simulink model "DATA_MTK_2"  (R2017a)
settings: Solver=ode1  StartTime=Times.Ts  StopTime=Times.Tsim  FixedStep=Times.Ts  RelTol=1e-3  EnableMultiTasking=on
values from neighbouring files (symbols this model uses):
  CL = 1    [Main_HydroVsData30min.m]
  WaveData = Init_waves_Data_V2(Time)    [Main_HydroVsData30min.m]
undefined symbols (not defined in the file or in its folder): Times, Turb, WEC
settings Model: Creator=FixnBock  LastModifiedBy=Temo
settings SolverCC: AlgebraicLoopSolver=LineSearch
settings DataIOCC: LimitDataPoints=on  SaveFormat=StructureWithTime
settings OptimizationCC: DefaultParameterBehavior=Inlined  LifeSpan=inf
settings DebuggingCC: AlgebraicLoopMsg=error  SFUnexpectedBacktrackingDiag=warning  SFNoUnconditionalDefaultTransitionDiag=warning  SFExecutionAtInitializationDiag=none
settings HardwareCC: ProdBitPerSizeT=32  ProdBitPerPtrDiffT=32  ProdWordSize=32  ProdHWDeviceType=Specified
settings ModelReferenceCC: PropagateSignalLabelsOutOfModel=off
settings RTWCC: TemplateMakefile=RTW.MSVCBuild  Description=Create Visual C/C++ Solution File for Simulink Coder
settings GRTTargetCC: TargetLangStandard=C89/C90 (ANSI)
settings ConfigComp: CovMetricSettings=dw  CovHtmlReporting=on  CovSaveCumulativeToWorkspaceVar=on  CovSaveSingleToWorkspaceVar=on  CovExternalEMLEnable=off

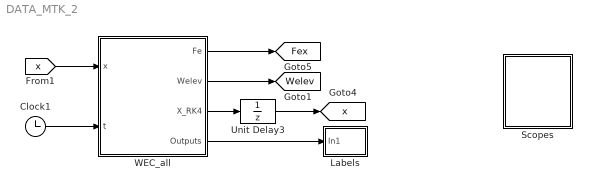
== system DATA_MTK_2 ==
  Clock1 : Clock
  Labels : Subsystem
  Scopes : Subsystem
  Unit Delay3 : UnitDelay  InitialCondition=WEC.X0  SampleTime=-1
  WEC_all : MATLAB Function  TreatAsAtomicUnit=on
  tag scope: Fex=global, Welev=global, x=global
  wires:
  Clock1/1 -> WEC_all/2(t)
  Unit Delay3/1 -> [x]
  [x] -> WEC_all/1(x)
  WEC_all/4(Outputs) -> Labels/1(In1)
  WEC_all/3(X_RK4) -> Unit Delay3/1
  WEC_all/1(Fe) -> [Fex]
  WEC_all/2(Welev) -> [Welev]

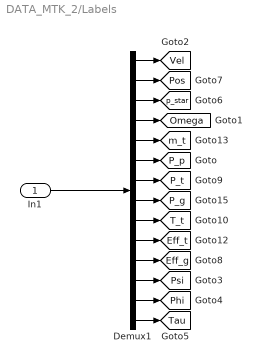
== system DATA_MTK_2/Labels ==
  In1 : Inport
  Demux1 : Demux  Outputs=14
  tag scope: Eff_g=global, Eff_t=global, Omega=global, P_g=global, P_p=global, P_t=global, Phi=global, Pos=global, Psi=global, T_t=global, Tau=global, Vel=global, m_t=global, p_star=global
  wires:
  Demux1/5 -> [m_t]
  Demux1/3 -> [p_star]
  Demux1/8 -> [P_g]
  Demux1/1 -> [Vel]
  Demux1/4 -> [Omega]
  Demux1/2 -> [Pos]
  Demux1/9 -> [T_t]
  Demux1/7 -> [P_t]
  Demux1/10 -> [Eff_t]
  Demux1/11 -> [Eff_g]
  Demux1/12 -> [Psi]
  Demux1/13 -> [Phi]
  Demux1/14 -> [Tau]
  Demux1/6 -> [P_p]
  In1/1 -> Demux1/1

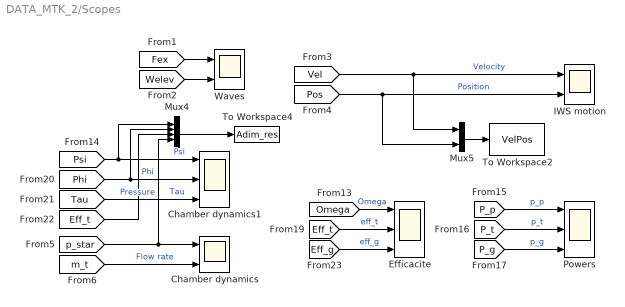
== system DATA_MTK_2/Scopes ==
  Chamber dynamics : Scope  NumInputPorts=2
  Chamber dynamics1 : Scope  NumInputPorts=3
  Efficacite : Scope  NumInputPorts=3
  IWS motion : Scope  NumInputPorts=2
  Mux4 : Mux
  Mux5 : Mux  Inputs=2
  Powers : Scope  NumInputPorts=3
  To Workspace2 : ToWorkspace  VariableName=VelPos  SampleTime=-1
      settings: Decimation=2
  To Workspace4 : ToWorkspace  VariableName=Adim_res  SampleTime=-1
      settings: Decimation=2
  Waves : Scope  NumInputPorts=2
  wires:
  [p_star] -> Mux4/4, Chamber dynamics/1  "Pressure"
  [m_t] -> Chamber dynamics/2  "Flow rate"
  [Welev] -> Waves/2
  [Fex] -> Waves/1
  [Psi] -> Mux4/1, Chamber dynamics1/1  "Psi"
  [Tau] -> Chamber dynamics1/3  "Tau"
  Mux4/1 -> To Workspace4/1
  [Eff_t] -> Mux4/3
  [Phi] -> Mux4/2, Chamber dynamics1/2  "Phi"
  [Vel] -> Mux5/1, IWS motion/1  "Velocity"
  [Pos] -> Mux5/2, IWS motion/2  "Position"
  Mux5/1 -> To Workspace2/1
  [Eff_t] -> Efficacite/2  "eff_t"
  [Eff_g] -> Efficacite/3  "eff_g"
  [P_g] -> Powers/3  "p_g"
  [P_t] -> Powers/2  "p_t"
  [P_p] -> Powers/1  "p_p"
  [Omega] -> Efficacite/1  "Omega"

== matlab function DATA_MTK_2/WEC_all ==
  data: x input size=24; t input; Fe output; WaveData parameter; WEC parameter; Turb parameter; Times parameter; CL parameter; Welev output; X_RK4 output; Outputs output
function [Fe,Welev,X_RK4,Outputs] = main(x,t,WaveData,WEC,Turb,Times,CL)

Ts = Times.Ts;

[Fexc,Welev] = resource(t,WaveData,WEC,Ts);
Fe = Fexc(3);

[X_RK4,Outputs] = fcn_rk4(t,x,Fexc,WEC,Turb,Ts,CL,Times);

end

function [Fe,welev] = resource(t,WaveData,WEC,Ts)
% Excitation force
smoother = min( 1.0 /  30 * t, 1.0 );
Fe_1  = smoother * WaveData.Wam .* WEC.Fint(1,:) * cos(WaveData.w_discr * (t+Ts) + WEC.Fint(2,:) + WaveData.Wpha)';    
Fe_k  = smoother * WaveData.Wam .* WEC.Fint(1,:) * cos(WaveData.w_discr * (t)    + WEC.Fint(2,:) + WaveData.Wpha)';    
Fe_05 = 0.5 * (Fe_1 + Fe_k);
% Wave elevation
welev = sum(WaveData.Wam * cos(WaveData.w_discr * t + WaveData.Wpha)');
 
Fe = [Fe_1, Fe_05, Fe_k];
end 

function [X_RK4,Outputs] = fcn_rk4(t,x,u,WEC,Turb,Ts,CL,Times)

Fexc_1  = u(1);
Fexc_05 = u(2);
Fexc_k  = u(3);

k1 = fcn_int(t,x,Fexc_k, WEC, Turb,CL,Times)*Ts;
k2 = fcn_int(t,x+k1/2,Fexc_05, WEC, Turb,CL,Times)*Ts;
k3 = fcn_int(t,x+k2/2,Fexc_05, WEC, Turb,CL,Times)*Ts;
k4 = fcn_int(t,x+k3,Fexc_1, WEC, Turb,CL,Times)*Ts;

X_RK4 = x + (k1+2*k2+2*k3+k4)/6;

[Outputs] = fcn_out(t,X_RK4,WEC,Turb,CL,Times);
end

function x_dot  = fcn_int(t,x,u,WEC,Turb,CL,Times)

% Keeps real part of the state vector and imaginary for the radiation terms
x(1)=real(x(1));
x(2)=real(x(2));
x(3)=real(x(3));
x(4)=real(x(4));

% Get derivate form
x_dot =  WEC.A * x +  WEC.B * u;

% From the state vector
p_star = x(3);

t_interp = linspace(Times.Ts,Times.Tsim,length(Turb.Om_opt));
Omega = interp1(t_interp,Turb.Om_opt,t); %Omega  = x(4); 

u_v = 1;

% Turbine characteristics
Intg_fun = 1;
[P_p, P_t, T_t, Eff_t,m_t] = PTO_Turbine(p_star,Omega,u_v,Intg_fun,WEC,Turb,CL);
% Generator characteristics
%Loss_gen = 1;
%[P_g, T_res, Eff_g] = PTO_Generator(T_ctrl,Omega,Loss_gen,Turb);

% Volume variation
V   = ( WEC.h_ch - x(2)) *  WEC.S_iws;
dV  = - x(1) *  WEC.S_iws;

%Polytropic 
Kappa = 1/(1-(WEC.beta*Eff_t));
Beta = (Kappa-1)/Kappa;

% p*_dot
% x_dot(3) = - m_t *  WEC.c_at2 / (  WEC.p_at * V )*( p_star + 1.0 )^ WEC.GM1_G ...
%          -  WEC.gamma * ( p_star + 1.0 ) * dV / V;
x_dot(3)= (-Kappa *(p_star+1)*(dV/V)) ...
        - ((Kappa*(p_star+1)^(Beta))*(m_t/(WEC.rho_at*V))) ; 
    
% Omega_dot
%x_dot(4) = (T_t - T_res) / Turb.I; 
%x_dot(4) = Omega;

% Batch BeP
%if CL == 0, x_dot(4) = 0; end
end

function [Sys_out] = fcn_out(t,x,WEC,Turb,CL,Times)

% Initialise output vector size
Sys_out = zeros(14,1);
% U_ctrl  = zeros(4,1); 

% From the state vector
vel   = real(x(1));
pos   = real(x(2));
p_star = real(x(3));

t_interp = linspace(Times.Ts,Times.Tsim,length(Turb.Om_opt));
Omega = interp1(t_interp,Turb.Om_opt,t);
if isnan(Omega)
    Omega = 0;
end
%Omega  = real(x(4));

u_v = 1;

if CL
%     % Control vector
%     if Omega > Turb.Om_Tci
%         %T_ctrl = u_ctrl(3) * Omega ^u_ctrl(4);
%     else
%         %T_ctrl = 0;
%     end
%     u_v = u_ctrl(2);

    % Turbine characteristics
    Intg_fun = 0;
    [P_p, P_t, T_t, Eff_t,m_t,valve_pos,Psi,Phi,Tau] = PTO_Turbine(p_star,Omega,u_v,Intg_fun,WEC,Turb,CL);
    % Generator characteristics
    %Loss_gen = 1;
    %[P_g, T_res, Eff_g] = PTO_Generator(T_ctrl,Omega,Loss_gen,Turb);
else 
    %Omega = interp1(t,Turb.Om_opt); 
    %u_v = u_ctrl(2);
    Intg_fun = 0;
    [P_p, P_t, T_t, Eff_t,m_t,valve_pos,Psi,Phi,Tau] = PTO_Turbine(p_star,Omega,u_v,Intg_fun,WEC,Turb,0);
    P_g = 0; T_res = 0; Eff_g = 0;
end

% Outputs
Sys_out(1) = vel;
Sys_out(2) = pos;
Sys_out(3) = p_star;
Sys_out(4) = Omega;
Sys_out(5) = m_t;
Sys_out(6) = P_p;
Sys_out(7) = P_t;
Sys_out(8) = 0;%P_g;
Sys_out(9) = T_t;
Sys_out(10) = Eff_t; 
Sys_out(11) = 0;%Eff_g;
Sys_out(12) = Psi; 
Sys_out(13) = Phi;
Sys_out(14) = Tau;
end
